simulink model "digital_filter_implementation"  (R2022b)
settings: Solver=VariableStepAuto  StartTime=0.0  StopTime=10.0  RelTol=1e-3
settings Model: Creator=ianmoone  LastModifiedBy=ianmoone
settings OptimizationCC: DefaultParameterBehavior=Inlined  UseDivisionForNetSlopeComputation=on  GainParamInheritBuiltInType=on  UseFloatMulNetSlope=on  InlineInvariantSignals=on  PassReuseOutputArgsAs=Individual arguments  ZeroExternalMemoryAtStartup=off  ZeroInternalMemoryAtStartup=off  NoFixptDivByZeroProtection=on  EfficientFloat2IntCast=on  LifeSpan=1  OptimizeBlockOrder=speed  DifferentSizesBufferReuse=on  EfficientTunableParamExpr=on
settings DebuggingCC: ParameterTunabilityLossMsg=error
settings HardwareCC: ProdBitPerLong=64  ProdLongLongMode=on  ProdHWDeviceType=Intel->x86-64 (Mac OS X)
settings SFSimCC: MATLABDynamicMemAlloc=off
settings RTWCC: Description=Embedded Coder  SystemTargetFile=ert.tlc  TemplateMakefile=ert_default_tmf
settings CodeAppCC: ForceParamTrailComments=on  IgnoreCustomStorageClasses=off  OperatorAnnotations=on  SimulinkDataObjDesc=on  SFDataObjDesc=on  CustomSymbolStrGlobalVar=rt$N$M  CustomSymbolStrType=$N$M  CustomSymbolStrFcn=$N$M$F  CustomSymbolStrMacro=$N$M  InsertBlockDesc=on
settings ERTTargetCC: TargetLangStandard=C99 (ISO)  GenerateSampleERTMain=on  IncludeMdlTerminateFcn=off  CombineSignalStateStructs=on  SuppressErrorStatus=on  SupportAbsoluteTime=off  PurelyIntegerCode=on  SupportNonFinite=off  SupportComplex=off  InlinedParameterPlacement=NonHierarchical  ERTCustomFileTemplate=example_file_process.tlc  ERTFilePackagingFormat=CompactWithDataFile

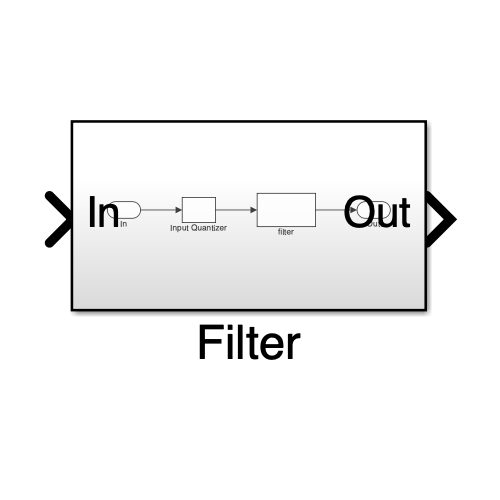
[thumbnail: Simulink's stored preview of the top-level diagram]
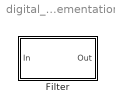
== system digital_filter_implementation ==
  Filter : Subsystem  Tag=BlockMethodSubSystem

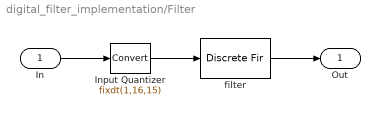
== system digital_filter_implementation/Filter ==
  In : Inport
  Input Quantizer : DataTypeConversion  OutDataTypeStr=fixdt(1,16,15)  RndMeth=Round
  filter : DiscreteFir  Coefficients=[-0.000919098208468256033 -0.00271769602659550002 -0.00248695275983231009 0.00366143838350709017 0.0136509252306624002 0.0173511659010932989 0.00766530619042168036 -0.00655471886964239994 -0.00769678403706536025 0.00610545942139436009 0.0138739157486354008 0.000350861728290910002 -0.0169089254366905015 -0.00890564274915867961 0.0174411295008548989 0.0207450445276099009 -0.0122964942519403 -0.034240865909578401 -0.00103452960557239991 0.0477903055208014974 0.0273630379148479992 -0.0593795188310465988 -0.0823070259292291023 0.0671869094328705063 0.310015177090251004 0.430047880343516986 0.310015177090251004 0.0671869094328705063 -0.0823070259292291023 -0.0593795188310465988 0.0273630379148479992 0.0477903055208014974 -0.00103452960557239991 -0.034240865909578401 -0.0122964942519403 0.0207450445276099009 0.0174411295008548989 -0.00890564274915867961 -0.0169089254366905015 0.000350861728290910002 0.0138739157486354008 0.00610545942139436009 -0.00769678403706536025 -0.00655471886964239994 0.00766530619042168036 0.0173511659010932989 0.0136509252306624002 0.00366143838350709017 -0.00248695275983231009 -0.00271769602659550002 -0.000919098208468256033]  InputProcessing=Columns as channels (frame based)  CoefDataTypeStr=fixdt(true,16,16)  ProductDataTypeStr=fixdt(true,31,31)  AccumDataTypeStr=fixdt(true,40,31)  OutDataTypeStr=fixdt(true,16,31)  SaturateOnIntegerOverflow=on
  Out : Outport
  wires:
  In/1 -> Input Quantizer/1
  Input Quantizer/1 -> filter/1
  filter/1 -> Out/1
